simulink model "LTS_GGV"  (R2024b)
settings: Solver=ode4  StartTime=0.0  StopTime=5  FixedStep=0.001  RelTol=1e-3
values from neighbouring files (symbols this model uses):
  Accelcmd = 0    [generate_GGV_LTS_GGV.m]
  Decelcmd = Brk    [generate_GGV_LTS_GGV.m]
  Omega0 = V0/Rw    [generate_GGV_LTS_GGV.m]
  Steer_rad = deg2rad(SteerDeg)    [generate_GGV_LTS_GGV.m]
libraries: autolibsharedcoupling x1, vehdynlibsteering x1, autolibmappedmotor x1, autolibshared x1
(part 1 of 2)
settings Model: Creator=ASUS  LastModifiedBy=ASUS
settings DataIOCC: SaveState=on  InspectSignalLogs=on

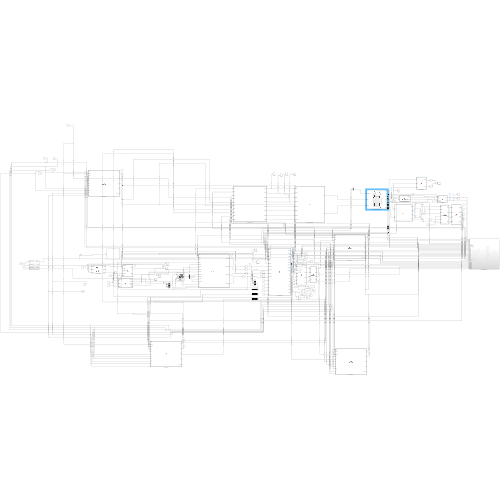
[thumbnail: Simulink's stored preview of the top-level diagram]
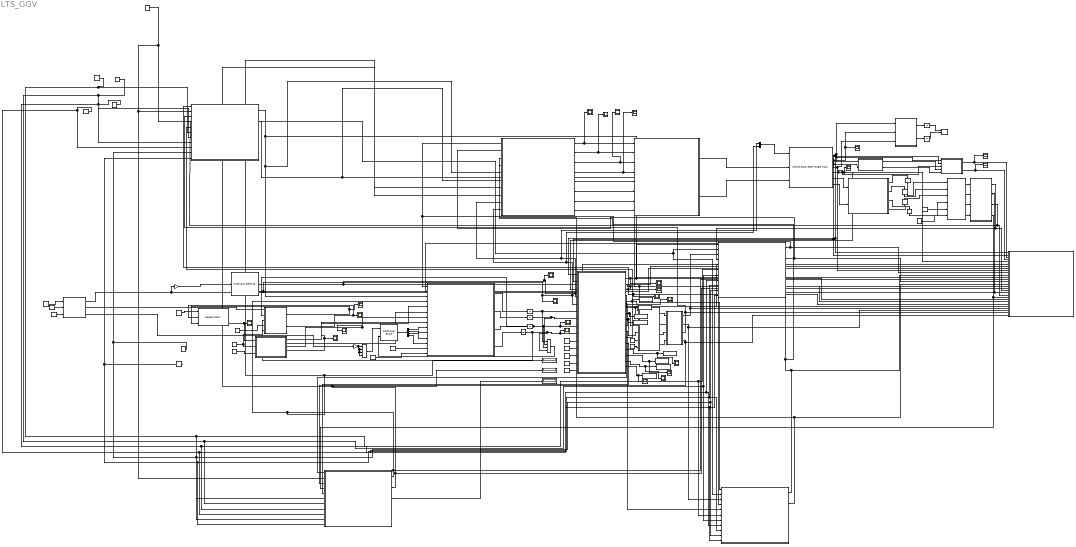
== system LTS_GGV ==
  "Accelaration " : MATLAB Function  TreatAsAtomicUnit=on
  Bodytoworld : MATLAB Function  TreatAsAtomicUnit=on
  Constant : Constant  Value=Steer_rad
  Constant1 : Constant  Value=0.10
  Constant10 : Constant  Value=0.001
  Constant11 : Constant  Value=0.08
  Constant12 : Constant  Value=0.03
  Constant13 : Constant  Value=0.001
  Constant14 : Constant  Value=Decelcmd
  Constant16 : Constant  Value=0.3
  Constant2 : Constant  Value=0.08
  Constant21 : Constant  Value=60
  Constant22 : Constant  Value=6
  Constant23 : Constant  Value=0.95
  Constant24 : Constant
  Constant3 : Constant  Value=0.30
  Constant31 : Constant  Value=0.8
  Constant32 : Constant  Value=0.8
  Constant33 : Constant  Value=1.2
  Constant34 : Constant  Value=1.2
  Constant35 : Constant  Value=0.3
  Constant4 : Constant
  Constant5 : Constant  Value=2.25e6
  Constant6 : Constant  Value=200
  Constant7 : Constant  Value=0
  Constant8 : Constant  Value=Accelcmd
  Constant9 : Constant
  Demux : Demux
  Disc Brake : autolibsharedcoupling/Rotational Brake  BrakeType=Disc  rotType=No inertia  extInfo=off  Iyy=1  br=1e-3  omegao=0  mu_static=0.4  mu_kinetic=0.35  disk_abore=0.02  Rm=0.08  num_pads=2  drum_abore=0.0508  drum_a=0.123  drum_c=0.212  drum_r=0.15  drum_theta1=0  drum_theta2=126  brake_p_bpt=[1 11.4736842105263 21.9473684210526 32.4210526315789 42.8947368421053 53.3684210526316 63.8421052631579 74.3157894736842 84.7894736842105 95.2631578947368 105.736842105263 116.210526315789 126.684210526316 137.157894736842 147.631578947368 158.105263157895 168.578947368421 179.052631578947 189.526315789474 200]  brake_n_bpt=[0 52.6315789473684 105.263157894737 157.894736842105 210.526315789474 263.157894736842 315.789473684211 368.421052631579 421.052631578947 473.684210526316 526.315789473684 578.947368421053 631.578947368421 684.210526315789 736.842105263158 789.473684210526 842.105263157895 894.736842105263 947.368421052632 1000]  f_brake_t=[43.4900602404453 42.5056030554862 41.5350898940194 40.5780454442085 39.6340111501808 38.7025443887544 37.7832176914519 36.8756180088306 35.9793460143796 35.0940154454303 34.2192524787115 33.3546951383474 32.4999927342521 31.6548053290159 30.8188032315107 29.991666515561 29.1730845621415 28.362755623661 27.5603864089927 26.765691687993;498.991217495636 487.695866636631 476.560505099801 465.579679307235 454.748127933653 444.060772460445 433.51270824929 423.099196101319 412.81565427025 402.657650900201 392.620896861006 382.701238955775 372.894653477208 363.197240090814 353.605216024701 344.114910546964 334.722759712992 325.425301366216 316.219170376863 307.10109410434;954.492374750826 932.886130217776 911.585920305583 890.581313170261 869.862244717126 849.419000532136 829.242198807128 809.322774193808 789.651962526121 770.221286354971 751.0225412433 732.047782773203 713.289314220164 694.739674852612 676.391628817892 658.238154578366 640.272434863842 622.48784710877 604.877954344734 587.436496520688;1409.99353200602 1378.07639379892 1346.61133551136 1315.58294703329 1284.9763615006 1254.77722860383 1224.97168936497 1195.5463522863 1166.48827078199 1137.78492180974 1109.42418562559 1081.39432659063 1053.68397496312 1026.28210961441 999.178041611083 972.361398609768 945.822110014692 919.550392851325 893.536738312604 867.771898937035;1865.49468926121 1823.26665738007 1781.63675071715 1740.58458089631 1700.09047828407 1660.13545667552 1620.7011799228 1581.76993037878 1543.32457903786 1505.34855726451 1467.82583000789 1430.74087040806 1394.07863570608 1357.82454437621 1321.96445440427 1286.48464264117 1251.37178516554 1216.61293859388 1182.19552228048 1148.10730135338;2320.9958465164 2268.45692096121 2216.66216592293 2165.58621475934 2115.20459506754 2065.49368474721 2016.43067048064 1967.99350847127 1920.16088729373 1872.91219271928 1826.22747439018 1780.08741422549 1734.47329644903 1689.36697913801 1644.75086719747 1600.60788667257 1556.92146031639 1513.67548433643 1470.85430624835 1428.44270376973;2776.49700377159 2713.64718454235 2651.68758112871 2590.58784862237 2530.31871185102 2470.8519128189 2412.16016103848 2354.21708656376 2296.9971955496 2240.47582817405 2184.62911877248 2129.43395804292 2074.86795719199 2020.9094138998 1967.53727999066 1914.73113070398 1862.47113546724 1810.73803007899 1759.51309021622 1708.77810618608;3231.99816102678 3158.8374481235 3086.71299633449 3015.58948248539 2945.43282863449 2876.21014089059 2807.88965159632 2740.44066465625 2673.83350380547 2608.03946362882 2543.03076315477 2478.78050186034 2415.26261793494 2352.4518486616 2290.32369278385 2228.85437473538 2168.02081061809 2107.80057582154 2048.17187418409 1989.11350860242;3687.49931828197 3604.02771170464 3521.73841154027 3440.59111634842 3360.54694541796 3281.56836896228 3203.61914215416 3126.66424274874 3050.66981206134 2975.60309908359 2901.43240753707 2828.12704567777 2755.6572786779 2683.9942834234 2613.11010557704 2542.97761876678 2473.57048576894 2404.8631215641 2336.83065815196 2269.44891101877;4143.00047553716 4049.21797528579 3956.76382674606 3865.59275021144 3775.66106220143 3686.92659703397 3599.34863271199 3512.88782084123 3427.50612031721 3343.16673453836 3259.83405191936 3177.4735894952 3096.05193942085 3015.5367181852 2935.89651837023 2857.10086279818 2779.12016091979 2701.92566730665 2625.48944211983 2549.78431343512;4598.50163279235 4494.40823886693 4391.78924195184 4290.59438407447 4190.77517898491 4092.28482510566 3995.07812326983 3899.11139893372 3804.34242857308 3710.73036999313 3618.23569630166 3526.82013331263 3436.44660016381 3347.079152947 3258.68293116342 3171.22410682959 3084.66983607064 2998.98821304921 2914.1482260877 2830.11971585147;5054.00279004754 4939.59850244808 4826.81465715762 4715.59601793749 4605.88929576838 4497.64305317735 4390.80761382767 4285.3349770262 4181.17873682896 4078.2940054479 3976.63734068395 3876.16667713006 3776.84126090677 3678.62158770879 3581.46934395661 3485.34735086099 ...(+2764 chars)]  aMode=2
      settings: LibrarySourceBlock=vehdynlibbrake/Disc Brake
  Display5 : Display
  Display6 : Display
  Display7 : Display
  "Force FWF and FWR " : MATLAB Function  TreatAsAtomicUnit=on
  Front_Left_tire : MATLAB Function  TreatAsAtomicUnit=on
  Front_Right_Tire : MATLAB Function  TreatAsAtomicUnit=on
  GGV Measurement : Subsystem
  Gain : Gain  Gain=8e+6
  Gain1 : Gain
  Integrator{,1..2,4} (4 alike) : Integrator  InitialCondition=Omega0
  Integrator3 : Integrator
  Integrator5 : Integrator
  Kinematic Steering : vehdynlibsteering/Kinematic Steering  StrgType=Ackerman  StrgRatioType=Constant  Loc=Front  NrmlFctr=0.01  TrckWdth=1.2  WhlBase=1.6  Db=0  StrgRng=deg2rad(25)  StrgAngBpts="[-6.2832   -5.0265   -3.7699   -2.5133   -1.2566         0    1.2566    2.5133    3.7699    5.0265    6.2832]"  StrgRatioTbl=|  StrgRatio=1  PctAckIn=off  PctAck=100  PctAckTbl=ones(1,11)*100  StrgArmLngth=0.1  RckCsLngth=0.5  TieRodLngth=0.248  D=0.2  PnnRadius=0.00085818  PnnRadiusTbl="[0.0055    0.0055    0.0056    0.0057    0.0058    0.0057    0.0057    0.0057    0.0056    0.0055    0.0055]"  RodLngth=0.1  ParaArmLngth=0.9  aMode=2
      | [13.5000   13.3750   13.2500   13.1250   13.0000   13.0000   13.0000   13.1250   13.2500   13.3750   13.5000
      | ]
  MATLAB Function : MATLAB Function  TreatAsAtomicUnit=on
  MATLAB Function1 : MATLAB Function  TreatAsAtomicUnit=on
  MATLAB Function2 : MATLAB Function  TreatAsAtomicUnit=on
  MATLAB Function3 : MATLAB Function  TreatAsAtomicUnit=on  SystemSampleTime=0.001
  MATLAB Function4 : MATLAB Function  TreatAsAtomicUnit=on
  MATLAB Function5 : MATLAB Function  TreatAsAtomicUnit=on  SystemSampleTime=0.001
  MATLAB Function6 : MATLAB Function  TreatAsAtomicUnit=on
  MATLAB Function7 : MATLAB Function  TreatAsAtomicUnit=on
  Mapped Motor : autolibmappedmotor/Mapped Motor  w_Tmax_bp_ext=w_Tmax_bp  Tmax_w_V_ext=Tmax_w_V  w_Tmin_bp_ext=w_Tmin_bp  Tmin_w_V_ext=Tmin_w_V  port_config=Speed  param_by=Maximum torque and power  w_t=[ 0 375 750 800 ]  T_t=[0.09 0.08 0.07 0]  torque_max=60  power_max=35000  SpreadsheetTqLimitsFileName=MotorCalibrationImportData.xlsx  Tmax_w_V=[0.09 0.09 0.09;0.08 0.08 0.08;0.07 0.07 0.07;0 0 0]  w_Tmax_bp=[ 0 375 750 800 ]  V_Tmax_bp=[500 750 900]  Tmin_w_V=[-0.09 -0.09 -0.09;-0.08 -0.08 -0.08;-0.07 -0.07 -0.07;0 0 0]  w_Tmin_bp=[ 0 375 750 800 ]  V_Tmin_bp=[500 750 900]  Tc=0.02  param_loss=Single efficiency measurement  SpreadsheetLossFileName=MotorCalibrationImportData.xlsx  SpreadsheetEffFileName=MotorCalibrationImportData.xlsx  eff=100  w_eff=375  T_eff=0.08  Piron=0  Pbase=0  w_eff_bp=[-8000 -4000 0 4000 8000]  T_eff_bp=[0 0.03 0.06 0.09]  Temp_eff_bp=[233.15 293.15 373.15]  V_eff_bp=[500 700 900]  losses_table=[1.49 1.67 2.21 3.10; 0.42 0.69 1.14 2.03; 0.06 0.24 0.78 1.68; 0.42 0.69 1.14 2.03; 1.49 1.67 2.21 3.10]  losses_table_3d=cat(3,1.05*[1.49 1.67 2.21 3.10; 0.42 0.69 1.14 2.03; 0.06 0.24 0.78 1.68; 0.42 0.69 1.14 2.03; 1.49 1.67 2.21 3.10],[1.49 1.67 2.21 3.10; 0.42 0.69 1.14 2.03; 0.06 0.24 0.78 1.68; 0.42 0.69 1.14 2.03; 1.49 1.67 2.21 3.10],1.03*[1.49 1.67 2.21 3.10; 0.42 0.69 1.14 2.03; 0.06 0.24 0.78 1.68; 0.42 0.69 1.14 2.03; 1.49 1.67 2.21 3.10])  losses_table_4d=cat(4,cat(3,[1.5645 0.441 0.063 0.441 1.5645;1.7535 0.7245 0.252 0.7245 1.7535;2.3205 1.197 0.819 1.197 2.3205;3.255 2.1315 1.764 2.1315 3.255],[1.5645 0.441 0.063 0.441 1.5645;1.7535 0.7245 0.252 0.7245 1.7535;2.3205 1.197 0.819 1.197 2.3205;3.255 2.1315 1.764 2.1315 3.255],[1.5645 0.441 0.063 0.441 1.5645;1.7535 0.7245 0.252 0.7245 1.7535;2.3205 1.197 0.819 1.197 2.3205;3.255 2.1315 1.764 2.1315 3.255]),cat(3,[1.49 0.42 0.06 0.42 1.49;1.67 0.69 0.24 0.69 1.67;2.21 1.14 0.78 1.14 2.21;3.1 2.03 1.68 2.03 3.1],[1.49 0.42 0.06 0.42 1.49;1.67 0.69 0.24 0.69 1.67;2.21 1.14 0.78 1.14 2.21;3.1 2.03 1.68 2.03 3.1],[1.49 0.42 0.06 0.42 1.49;1.67 0.69 0.24 0.69 1.67;2.21 1.14 0.78 1.14 2.21;3.1 2.03 1.68 2.03 3.1]),cat(3,[1.5347 0.4326 0.0618 0.4326 1.5347;1.7201 0.7107 0.2472 0.7107 1.7201;2.2763 1.1742 0.8034 1.1742 2.2763;3.193 2.0909 1.7304 2.0909 3.193],[1.5347 0.4326 0.0618 0.4326 1.5347;1.7201 0.7107 0.2472 0.7107 1.7201;2.2763 1.1742 0.8034 1.1742 2.2763;3.193 2.0909 1.7304 2.0909 3.193],[1.5347 0.4326 0.0618 0.4326 1.5347;1.7201 0.7107 0.2472 0.7107 1.7201;2.2763 1.1742 0.8034 1.1742 2.2763;3.193 2.0909 1.7304 2.0909 3.193]))  efficiency_table=[95 95 95 95; 95 95 95 95; 95 95 95 95; 95 95 95 95; 95 95 95 95]  efficiency_table_3d=cat(3,90*ones(5,4),95*ones(5,4),92*ones(5,4))  efficiency_table_4d=cat(4,cat(3,90*ones(5,4)',90*ones(5,4)',90*ones(5,4)'),cat(3,95*ones(5,4)',95*ones(5,4)',95*ones(5,4)'),cat(3,92*ones(5,4)',92*ones(5,4)',92*ones(5,4)'))  J=5e-6  b=1e-5  omega_o=0  T_t_extended=[0 0.07 0.08 0.09 0.08 0.07 0]  w_t_extended=[-800 -750 -375 0 375 750 800]  KLossIron=0  KLossCopper=0  x_w_eff_vec=[-8000 -4000 0 4000 8000]  x_T_eff_vec=[-0.09 -0.06 -0.03 0 0.03 0.06 0.09]  x_tmp_eff_vec=[233.15 293.15 373.15]  x_V_eff_vec=[500 700 900]  x_losses_mat=[3.1 2.21 1.67 1.49 1.67 2.21 3.1;2.03 1.14 0.69 0.42 0.69 1.14 2.03;1.68 0.78 0.24 0.06 0.24 0.78 1.68;2.03 1.14 0.69 0.42 0.69 1.14 2.03;3.1 2.21 1.67 1.49 1.67 2.21 3.1]  x_losses_mat_3d=cat(3,[3.255 2.3205 1.7535 1.5645 1.7535 2.3205 3.255;2.1315 1.197 0.7245 0.441 0.7245 1.197 2.1315;1.764 0.819 0.252 0.063 0.252 0.819 1.764;2.1315 1.197 0.7245 0.441 0.7245 1.197 2.1315;3.255 2.3205 1.7535 1.5645 1.7535 2.3205 3.255],[3.1 2.21 1.67 1.49 1.67 2.21 3.1;2.03 1.14 0.69 0.42 0.69 1.14 2.03;1.68 0.78 0.24 0.06 0.24 0.78 1.68;2.03 1.14 0.69 0.42 0.69 1.14 2.03;3.1 2.21 1.67 1.49 1.67 2.21 3.1],[3.193 2.2763 1.7201 1.5347 1.7201 2.2763 3.193;2.0909 1.1742 0.7107 0.4326 0.7107 1.1742 2.0909;1.7304 0.8034 0.2472 0.0618 0.2472 0.8034 1.7304;2.0909 1.1742 0.7107 0.4326 0.7107 1.1742 2.0909;3.193 2.2763 1.7201 1.5347 1.7201 2.2763 3.193])  x_losses_mat_4d=cat(4,cat(3,[1.5645 0.441 0.063 0.441 1.5645;1.7535 0.7245 0.252 0.7245 1.7535;2.3205 1.197 0.819 1.197 2.3205;3.255 2.1315 1.764 2.1315 3.255],[1.5645 0.441 0.063 0.441 1.5645;1.7535 0.7245 0.252 0.7245 1.7535;2.3205 1.197 0.819 1.197 2.3205;3.255 2.1315 1.764 2.1315 3.255],[1.5645 0.441 0.063 0.441 1.5645;1.7535 0.7245 0.252 0.7245 1.7535;2.3205 1.197 0.819 1.197 2.3205;3.255 2.1315 1.764 2.1315 3.255]),cat(3,[1.49 0.42 0.06 0.42 1.49;1.67 0.69 0.24 0.69 1.67;2.21 1.14 0.78 1.14 2.21;3.1 2.03 1.68 2.03 3.1],[1.49 0.42 0.06 0.42 1.49;1.67 0.69 0.24 0.69 1.67;2.21 1.14 0.78 1.14 2.21;3.1 2.03 1.68 2.03 3.1],[1.49 0.42 0.06 0.42 1.49;1.67 0.69 0.24 0.69 1.67;2.21 1.14 0.78 1.14 2.21;3.1 2.03 1.68 2.03 3.1]),cat(3,[1.5347 0.4326 0.0618 0.4326 1.5347;1.7201 0.7107 0.2472 0.7107 1.7201;2.2763 1.1742 0.8034 1.1742 2.2763;3.193 2.0909 1.7304 2.0909 3.193],[1.5347 0.4326 0.0618 0.4326 1.5347;1.7201 0.7107 0.2472 0.7107 1.7201;2.2763 1.1742 0.8034 1.1742 2.2763;3.193 2.0909 1.7304 2.0909 3.193],[1.5347 0.4326 0.0618 0.4326 1.5347;1.7201 0.7107 0.2472 0.7107 1.7201;2.2763 1.1742 0.8034 1.1742 2.2763;3.193 2.0909 1.7304 2.0909 3.193]))  CalLossMapData={}  CalLossWithTempMapData={}  aMode=2  RefBlkName='autolibmappedmotor/Mapped Motor'
      settings: LibrarySourceBlock=vdynlib/Powertrain/Propulsion/Mapped Motor
  Memory{,1..3} (4 alike) : Memory  InitialCondition=735.38
  Motor torque : Scope
  Mtr speed : Scope
  Mux : Mux  Inputs=2
  Omega RL : Scope
  Omega RR : Scope
  R : Scope
  "Rear_left tire " : MATLAB Function  TreatAsAtomicUnit=on
  Rear_right_tire : MATLAB Function  TreatAsAtomicUnit=on
  Scope{,1..9} (10 alike) : Scope
  Subsystem : Subsystem
  Tdrive RL : Scope
  Tdrive RR : Scope
  To Workspace1 : ToWorkspace  VariableName=VywFL  SampleTime=-1
      settings: Decimation=10
  To Workspace2 : ToWorkspace  VariableName=VxwFR  SampleTime=-1
      settings: Decimation=10
  To Workspace27 : ToWorkspace  VariableName=VxwFL  SampleTime=-1
      settings: Decimation=10
  To Workspace3 : ToWorkspace  VariableName=VywFR  SampleTime=-1
      settings: Decimation=10
  To Workspace4 : ToWorkspace  VariableName=kappaFL  SampleTime=-1
      settings: Decimation=10
  To Workspace5 : ToWorkspace  VariableName=kappaFR  SampleTime=-1
      settings: Decimation=10
  To Workspace6 : ToWorkspace  VariableName=kappaRL  SampleTime=-1
      settings: Decimation=10
  To Workspace7 : ToWorkspace  VariableName=kappaRR  SampleTime=-1
      settings: Decimation=10
  Trq commmand : Scope
  UY : Scope
  Vector Concatenate : Concatenate  NumInputs=4
  Vector Concatenate1 : Concatenate  NumInputs=4
  Vehicle Body 3DOF Dual Track : autolibshared/Vehicle Body 3DOF Single Track  trackMode=Dual  inputMode=External forces  frontSteerMode=on  rearSteerMode=off  windMode=off  muMode=off  extFMode=off  extMMode=off  htchFMode=off  htchMMode=off  extXo=off  extpsio=off  extxdoto=off  extro=off  extYo=off  extTamb=off  extydoto=off  aMode=2  NF=2  NR=2  m=300  a=0.8  b=0.8  h=0.3  dh=1  hh=0.2  X_o=0  xdot_o=V0  CalphaMode=off  sigmaMode=on  d=0  hl=0  w=[1.2,1.2]  Cy_f=12e3  Cy_r=11e3  sigma_f=.1  sigma_r=.1  alpha_f_brk=[-.1 .1]  Cy_f_data=[-9e3 9e3]  alpha_r_brk=[-.1 .1]  Cy_r_data=[-9e3 9e3]  Y_o=0  ydot_o=0  Izz=120  psi_o=0  r_o=0  Af=0  Cd=0  Cl=0  Cpm=0  beta_w=[0 0.01:0.01:0.3]  Cs=[0:0.03:0.9]  Cym=[0 1e-6:0.01:0.3]  Pabs=101325  Tair=273  g=9.81  mu=1  xdot_tol=.01  Fznom=5000  Fxtire_sat=7e4  Fytire_sat=7e4  longOff=0  latOff=0  vertOff=0  wrapAng=off
      settings: LibrarySourceBlock=vehdynlibeom/Vehicle Body 3DOF Dual Track
  VehicleVelocityDerivative : MATLAB Function  TreatAsAtomicUnit=on
  Wheel kinematics : MATLAB Function  TreatAsAtomicUnit=on
  XY Graph : Record  FileSettingsInternal="{\"entries\":[{\"content\":{\"excelSettings\":{\"content\":{},\"type\":\"Streamout.ExcelSettings\"}},\"type\":\"Streamout.FileSettingStorage\",\"uuid\":\"\"}],\"packageUris\":[\"http:\\/\\/schema.mathworks.com\\/mf0\\/streamout_blocks\\/R2020a\"],\"version\":\"1.0\"}"  Layout=[1 1]  SignalsInternal="{\"entries\":[{\"content\":{\"signals\":[{\"content\":{\"blockPath\":[],\"dimensions\":[1],\"domain\":\"\",\"lineColor\":\"#edb120\",\"lineWidth\":2,\"port\":1,\"sid\":[\"\"],\"signalID\":1,\"signalName\":\"X_sim\"},\"type\":\"RecordBlkView.Signal\",\"uuid\":\"\"},{\"content\":{\"blockPath\":[],\"dimensions\":[1],\"domain\":\"\",\"lineColor\":\"#7e2f8e\",\"lineWidth\":2,\"port\":2,\"sid\":[\"\"],\"signalID\":2,\"signalName\":\"Y_sim\"},\"type\":\"RecordBlkView.Signal\",\"uuid\":\"\"}]},\"type\":\"RecordBlkView.InputSignals\",\"uuid\":\"\"}],\"packageUris\":[\"http:\\/\\/schema.mathworks.com\\/mf0\\/streamout_blocks\\/R2020a\"],\"version\":\"1.0\"}"  VisualizationBindings="{\"xyplotplugin\":{\"info\":[{\"series\":[],\"subplotID\":1}]}}"  CompatibilityTag=XY
  fx fl : Scope
  fxfr : Scope
  fyfl : Scope
  fyfr : Scope
  "left angle " : Scope
  "right angle " : Scope
  "wheel to vehicle " : MATLAB Function  TreatAsAtomicUnit=on
  wires:
  Mux/1 -> Vehicle Body 3DOF Dual Track/1
  Integrator4/1 -> Vector Concatenate/4, Omega RR/1, Wheel kinematics/9(omegaRR), MATLAB Function6/3(omegaRR)
  MATLAB Function4/1(kFLs) -> GGV Measurement/26(KappaFL), Front_Left_tire/3(kappa)
  "Force FWF and FWR "/2(FwR) -> Vehicle Body 3DOF Dual Track/3
  Vehicle Body 3DOF Dual Track/7 -> MATLAB Function/2(FzR)
  Integrator2/1 -> Omega RL/1, Wheel kinematics/8(omegaRL), Vector Concatenate/3, MATLAB Function6/2(omegaRL)
  MATLAB Function4/2(kFRs) -> GGV Measurement/27(KappaFR), Front_Right_Tire/3(kappa)
  MATLAB Function4/3(kRLs) -> GGV Measurement/28(KappaRL), "Rear_left tire "/3(kappa)
  MATLAB Function4/4(kRRs) -> GGV Measurement/29(KappaRR), Rear_right_tire/3(kappa)
  Integrator/1 -> Vector Concatenate/1, Wheel kinematics/6(omegaFL)
  Vehicle Body 3DOF Dual Track/4 -> Bodytoworld/3(psi), GGV Measurement/9(PSI)
  Vehicle Body 3DOF Dual Track/3 -> "Accelaration "/2(ydot), Bodytoworld/2(ydot), UY/1, Wheel kinematics/2(Uy), GGV Measurement/2(Vy), VehicleVelocityDerivative/2(Uy)
  Vehicle Body 3DOF Dual Track/2 -> VehicleVelocityDerivative/1(Ux), "Accelaration "/1(xdot), Bodytoworld/1(xdot), GGV Measurement/1(Vx), Wheel kinematics/1(Ux)
  Vehicle Body 3DOF Dual Track/5 -> "Accelaration "/3(r), Wheel kinematics/3(r), R/1, GGV Measurement/5(r)
  Vehicle Body 3DOF Dual Track/6 -> MATLAB Function/1(FzF)
  Kinematic Steering/3 -> GGV Measurement/8(front-right steer), "right angle "/1, Wheel kinematics/5(deltaFR), Mux/2, "wheel to vehicle "/10(deltaFR)
  Front_Left_tire/2(Fy) -> "wheel to vehicle "/2(FyFL), GGV Measurement/14(FyFL)
  "wheel to vehicle "/4(FyVehFR) -> fyfr/1, "Force FWF and FWR "/4(FyVehFR)
  Constant6/1 -> "Rear_left tire "/11(n), Front_Right_Tire/11(n), Front_Left_tire/11(n), Rear_right_tire/11(n)
  Rear_right_tire/2(Fy) -> GGV Measurement/17(FyRR), Display6/1, "wheel to vehicle "/8(FyRR)
  Constant16/1 -> MATLAB Function1/13(Rw)
  Wheel kinematics/12(VcRR) -> Rear_right_tire/5(Vc)
  Constant34/1 -> Wheel kinematics/13(tr)
  Integrator1/1 -> Vector Concatenate/2, Wheel kinematics/7(omegaFR)
  Constant5/1 -> Front_Left_tire/10(cp), Front_Right_Tire/10(cp), Rear_right_tire/10(cp), "Rear_left tire "/10(cp)
  MATLAB Function1/2(omegaDotFR) -> Integrator1/1
  Front_Right_Tire/2(Fy) -> GGV Measurement/15(FyFR), "wheel to vehicle "/4(FyFR)
  "Rear_left tire "/1(Fx) -> GGV Measurement/12(FxRL), MATLAB Function1/3(FxRL), "wheel to vehicle "/5(FxRL)
  Constant35/1 -> Wheel kinematics/14(Rw)
  Constant32/1 -> Wheel kinematics/11(lr)
  MATLAB Function1/4(omegaDotRR) -> Integrator4/1
  Front_Right_Tire/1(Fx) -> GGV Measurement/11(FxFR), MATLAB Function1/2(FxFR), "wheel to vehicle "/3(FxFR)
  Constant3/1 -> "Rear_left tire "/8(re), Front_Left_tire/8(re), Front_Right_Tire/8(re), Rear_right_tire/8(re)
  "wheel to vehicle "/6(FyVehRL) -> "Force FWF and FWR "/6(FyVehRL)
  Wheel kinematics/9(VcFL) -> Front_Left_tire/5(Vc)
  Constant4/1 -> "Rear_left tire "/9(mu0), Front_Left_tire/9(mu0), Front_Right_Tire/9(mu0), Rear_right_tire/9(mu0)
  Constant7/1 -> Front_Right_Tire/2(gamma), Front_Left_tire/2(gamma), Rear_right_tire/2(gamma), "Rear_left tire "/2(gamma)
  "wheel to vehicle "/1(FxVehFL) -> fx fl/1, "Force FWF and FWR "/1(FxVehFL)
  "wheel to vehicle "/3(FxVehFR) -> fxfr/1, "Force FWF and FWR "/3(FxVehFR)
  Rear_right_tire/3(Mz) -> Display7/1
  Front_Left_tire/1(Fx) -> GGV Measurement/10(FxFL), MATLAB Function1/1(FxFL), "wheel to vehicle "/1(FxFL)
  MATLAB Function1/1(omegaDotFL) -> Integrator/1
  Wheel kinematics/3(alphaRL) -> Scope2/1, GGV Measurement/24(AlphaRL), "Rear_left tire "/1(alpha)
  Rear_right_tire/1(Fx) -> GGV Measurement/13(FxRR), MATLAB Function1/4(FxRR), Display5/1, "wheel to vehicle "/7(FxRR)
  Constant1/1 -> "Rear_left tire "/6(a), Front_Left_tire/6(a), Front_Right_Tire/6(a), Rear_right_tire/6(a)
  Wheel kinematics/11(VcRL) -> "Rear_left tire "/5(Vc)
  Kinematic Steering/2 -> GGV Measurement/7(front-left steer), Wheel kinematics/4(deltaFL), Mux/1, "wheel to vehicle "/9(deltaFL), "left angle "/1
  Constant31/1 -> Wheel kinematics/10(lf)
  MATLAB Function1/3(omegaDotRL) -> Integrator2/1
  Wheel kinematics/4(alphaRR) -> Scope3/1, GGV Measurement/25(AlphaRR), Rear_right_tire/1(alpha)
  "wheel to vehicle "/5(FxVehRL) -> "Force FWF and FWR "/5(FxVehRL)
  Wheel kinematics/1(alphaFL) -> Scope/1, GGV Measurement/22(AlphaFL), Front_Left_tire/1(alpha)
  Constant2/1 -> "Rear_left tire "/7(b), Front_Left_tire/7(b), Front_Right_Tire/7(b), Rear_right_tire/7(b)
  Wheel kinematics/10(VcFR) -> Front_Right_Tire/5(Vc)
  "wheel to vehicle "/8(FyVehRR) -> "Force FWF and FWR "/8(FyVehRR)
  Constant33/1 -> Wheel kinematics/12(tf)
  Constant9/1 -> MATLAB Function1/14(Iw)
  "wheel to vehicle "/7(FxVehRR) -> "Force FWF and FWR "/7(FxVehRR)
  "wheel to vehicle "/2(FyVehFL) -> fyfl/1, "Force FWF and FWR "/2(FyVehFL)
  Wheel kinematics/2(alphaFR) -> Scope1/1, GGV Measurement/23(AlphaFR), Front_Right_Tire/1(alpha)
  "Rear_left tire "/2(Fy) -> GGV Measurement/16(FyRL), "wheel to vehicle "/6(FyRL)
  "Force FWF and FWR "/1(FwF) -> Vehicle Body 3DOF Dual Track/2
  MATLAB Function/4(FzRR) -> Memory3/1
  MATLAB Function/1(FzFL) -> Memory/1
  MATLAB Function/2(FzFR) -> Memory2/1
  MATLAB Function/3(FzRL) -> Memory1/1
  Memory/1 -> MATLAB Function2/1(FzFL)
  Memory1/1 -> MATLAB Function2/3(FzRL)
  Memory2/1 -> MATLAB Function2/2(FzFR)
  Memory3/1 -> MATLAB Function2/4(FzRR)
  MATLAB Function3/3(FzRLs) -> "Rear_left tire "/4(Fz), GGV Measurement/20(FzRL)
  MATLAB Function3/1(FzFLs) -> GGV Measurement/18(FzFL), Front_Left_tire/4(Fz)
  MATLAB Function3/2(FzFRs) -> GGV Measurement/19(FzFR), Front_Right_Tire/4(Fz)
  MATLAB Function3/4(FzRRs) -> Rear_right_tire/4(Fz), GGV Measurement/21(FzRR)
  Constant10/1 -> MATLAB Function2/5(dt)
  Constant11/1 -> MATLAB Function2/6(tau)
  MATLAB Function2/1(FzFLf) -> MATLAB Function3/1(FzFL)
  MATLAB Function2/2(FzFRf) -> MATLAB Function3/2(FzFR)
  MATLAB Function2/3(FzRLf) -> MATLAB Function3/3(FzRL)
  MATLAB Function2/4(FzRRf) -> MATLAB Function3/4(FzRR)
  Wheel kinematics/8(kappaRR) -> To Workspace7/1, MATLAB Function5/4(kRR)
  Wheel kinematics/6(kappaFR) -> To Workspace5/1, MATLAB Function5/2(kFR)
  Wheel kinematics/5(kappaFL) -> To Workspace4/1, MATLAB Function5/1(kFL)
  Disc Brake/1 -> Demux/1
  MATLAB Function5/1(kFLf) -> MATLAB Function4/1(kFL)
  MATLAB Function5/2(kFRf) -> MATLAB Function4/2(kFR)
  MATLAB Function5/3(kRLf) -> MATLAB Function4/3(kRL)
  MATLAB Function5/4(kRRf) -> MATLAB Function4/4(kRR)
  Constant12/1 -> MATLAB Function5/6(tau)
  Constant13/1 -> MATLAB Function5/5(dt)
  Mapped Motor/3 -> MATLAB Function7/1(MtrTrq), Motor torque/1
  Constant21/1 -> MATLAB Function6/4(TmotorMax)
  Constant22/1 -> MATLAB Function7/2(Ndiff), MATLAB Function6/5(Ndiff)
  Constant23/1 -> MATLAB Function7/3(etaDiff)
  MATLAB Function6/1(TrqCmd) -> Mapped Motor/3, Trq commmand/1
  MATLAB Function6/2(MtrSpd) -> Mtr speed/1, Mapped Motor/2
  Constant24/1 -> Mapped Motor/1
  MATLAB Function7/1(TdriveFL) -> MATLAB Function1/5(TdriveFL)
  MATLAB Function7/2(TdriveFR) -> MATLAB Function1/6(TdriveFR)
  MATLAB Function7/3(TdriveRL) -> MATLAB Function1/7(TdriveRL), Tdrive RL/1
  MATLAB Function7/4(TdriveRR) -> MATLAB Function1/8(TdriveRR), Tdrive RR/1
  Vector Concatenate/1 -> Disc Brake/2
  Gain/1 -> Vector Concatenate1/4, Vector Concatenate1/3, Vector Concatenate1/2, Vector Concatenate1/1
  Vector Concatenate1/1 -> Disc Brake/1
  Demux/1 -> MATLAB Function1/9(TbrakeFL)
  Demux/2 -> MATLAB Function1/10(TbrakeFR)
  Demux/3 -> MATLAB Function1/11(TbrakeRL)
  Demux/4 -> MATLAB Function1/12(TbrakeRR)
  Bodytoworld/1(Xdot_w) -> Integrator3/1
  Bodytoworld/2(Ydot_w) -> Integrator5/1
  Integrator3/1 -> XY Graph/1  "X_sim"
  Integrator5/1 -> XY Graph/2  "Y_sim"
  Gain1/1 -> Kinematic Steering/1
  VehicleVelocityDerivative/1(Ux_dot) -> "Accelaration "/4(xdot_deriv)
  VehicleVelocityDerivative/2(Uy_dot) -> "Accelaration "/5(ydot_deriv)
  "Accelaration "/2(ay_G) -> Scope9/1, GGV Measurement/4(Ay)
  "Accelaration "/1(ax_G) -> Scope8/1, GGV Measurement/3(Ax)
  Subsystem/1(SteerCmd) -> GGV Measurement/6(steer_cmd), Gain1/1
  Subsystem/2(Accel) -> MATLAB Function6/1(throttleCmd)
  Subsystem/3(Decel) -> Gain/1
  Wheel kinematics/13(VxwFL) -> Scope4/1, To Workspace27/1
  Wheel kinematics/14(VywFL) -> Scope5/1, To Workspace1/1
  Wheel kinematics/15(VxwFR) -> Scope6/1, To Workspace2/1
  Wheel kinematics/16(VywFR) -> Scope7/1, To Workspace3/1
  Constant/1 -> Subsystem/1(" SteerCmd_GGV")
  Constant8/1 -> Subsystem/2(AccelCmd_GGV)
  Constant14/1 -> Subsystem/3(DecelCmd_GGV)
  Wheel kinematics/7(kappaRL) -> To Workspace6/1, MATLAB Function5/3(kRL)

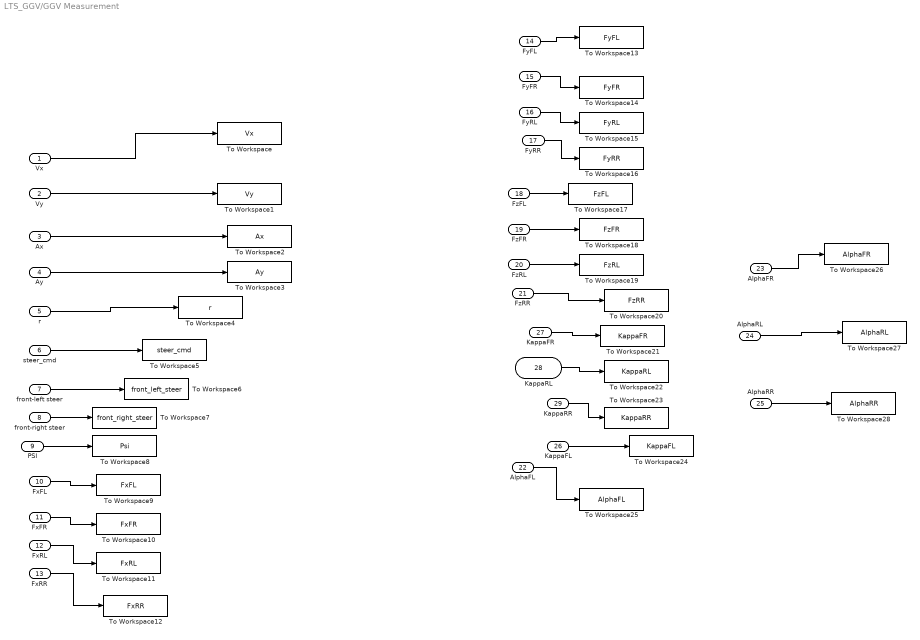
== system LTS_GGV/GGV Measurement ==
  Vx : Inport
  Vy : Inport  Port=2
  Ax : Inport  Port=3
  Ay : Inport  Port=4
  r : Inport  Port=5
  steer_cmd : Inport  Port=6
  front-left steer : Inport  Port=7
  front-right steer : Inport  Port=8
  PSI : Inport  Port=9
  FxFL : Inport  Port=10
  FxFR : Inport  Port=11
  FxRL : Inport  Port=12
  FxRR : Inport  Port=13
  FyFL : Inport  Port=14
  FyFR : Inport  Port=15
  FyRL : Inport  Port=16
  FyRR : Inport  Port=17
  FzFL : Inport  Port=18
  FzFR : Inport  Port=19
  FzRL : Inport  Port=20
  FzRR : Inport  Port=21
  AlphaFL : Inport  Port=22
  AlphaFR : Inport  Port=23
  AlphaRL : Inport  Port=24
  AlphaRR : Inport  Port=25
  KappaFL : Inport  Port=26
  KappaFR : Inport  Port=27
  KappaRL : Inport  Port=28
  KappaRR : Inport  Port=29
  To Workspace : ToWorkspace  VariableName=Vx  SampleTime=-1
      settings: Decimation=10
  To Workspace1 : ToWorkspace  VariableName=Vy  SampleTime=-1
      settings: Decimation=10
  To Workspace10 : ToWorkspace  VariableName=FxFR  SampleTime=-1
      settings: Decimation=10
  To Workspace11 : ToWorkspace  VariableName=FxRL  SampleTime=-1
      settings: Decimation=10
  To Workspace12 : ToWorkspace  VariableName=FxRR  SampleTime=-1
      settings: Decimation=10
  To Workspace13 : ToWorkspace  VariableName=FyFL  SampleTime=-1
      settings: Decimation=10
  To Workspace14 : ToWorkspace  VariableName=FyFR  SampleTime=-1
      settings: Decimation=10
  To Workspace15 : ToWorkspace  VariableName=FyRL  SampleTime=-1
      settings: Decimation=10
  To Workspace16 : ToWorkspace  VariableName=FyRR  SampleTime=-1
      settings: Decimation=10
  To Workspace17 : ToWorkspace  VariableName=FzFL  SampleTime=-1
      settings: Decimation=10
  To Workspace18 : ToWorkspace  VariableName=FzFR  SampleTime=-1
      settings: Decimation=10
  To Workspace19 : ToWorkspace  VariableName=FzRL  SampleTime=-1
      settings: Decimation=10
  To Workspace2 : ToWorkspace  VariableName=Ax  SampleTime=-1
      settings: Decimation=10
  To Workspace20 : ToWorkspace  VariableName=FzRR  SampleTime=-1
      settings: Decimation=10
  To Workspace21 : ToWorkspace  VariableName=KappaFR  SampleTime=-1
      settings: Decimation=10
  To Workspace22 : ToWorkspace  VariableName=KappaRL  SampleTime=-1
      settings: Decimation=10
  To Workspace23 : ToWorkspace  VariableName=KappaRR  SampleTime=-1
      settings: Decimation=10
  To Workspace24 : ToWorkspace  VariableName=KappaFL  SampleTime=-1
      settings: Decimation=10
  To Workspace25 : ToWorkspace  VariableName=AlphaFL  SampleTime=-1
      settings: Decimation=10
  To Workspace26 : ToWorkspace  VariableName=AlphaFR  SampleTime=-1
      settings: Decimation=10
  To Workspace27 : ToWorkspace  VariableName=AlphaRL  SampleTime=-1
      settings: Decimation=10
  To Workspace28 : ToWorkspace  VariableName=AlphaRR  SampleTime=-1
      settings: Decimation=10
  To Workspace3 : ToWorkspace  VariableName=Ay  SampleTime=-1
      settings: Decimation=10
  To Workspace4 : ToWorkspace  VariableName=r  SampleTime=-1
      settings: Decimation=10
  To Workspace5 : ToWorkspace  VariableName=steer_cmd  SampleTime=-1
      settings: Decimation=10
  To Workspace6 : ToWorkspace  VariableName=front_left_steer  SampleTime=-1
      settings: Decimation=10
  To Workspace7 : ToWorkspace  VariableName=front_right_steer  SampleTime=-1
      settings: Decimation=10
  To Workspace8 : ToWorkspace  VariableName=Psi  SampleTime=-1
      settings: Decimation=10
  To Workspace9 : ToWorkspace  VariableName=FxFL  SampleTime=-1
      settings: Decimation=10
  wires:
  Vx/1 -> To Workspace/1
  Vy/1 -> To Workspace1/1
  Ax/1 -> To Workspace2/1
  Ay/1 -> To Workspace3/1
  r/1 -> To Workspace4/1
  steer_cmd/1 -> To Workspace5/1
  front-left steer/1 -> To Workspace6/1
  front-right steer/1 -> To Workspace7/1
  PSI/1 -> To Workspace8/1
  FxFL/1 -> To Workspace9/1
  FxFR/1 -> To Workspace10/1
  FxRL/1 -> To Workspace11/1
  FxRR/1 -> To Workspace12/1
  FyFL/1 -> To Workspace13/1
  FyFR/1 -> To Workspace14/1
  FyRL/1 -> To Workspace15/1
  FyRR/1 -> To Workspace16/1
  FzFL/1 -> To Workspace17/1
  FzFR/1 -> To Workspace18/1
  FzRL/1 -> To Workspace19/1
  FzRR/1 -> To Workspace20/1
  KappaFR/1 -> To Workspace21/1
  KappaRL/1 -> To Workspace22/1
  KappaRR/1 -> To Workspace23/1
  KappaFL/1 -> To Workspace24/1
  AlphaFL/1 -> To Workspace25/1
  AlphaFR/1 -> To Workspace26/1
  AlphaRL/1 -> To Workspace27/1
  AlphaRR/1 -> To Workspace28/1

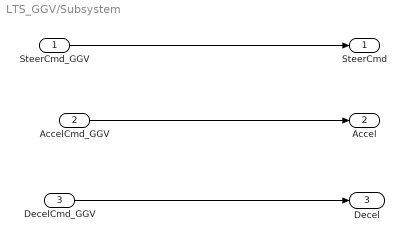
== system LTS_GGV/Subsystem ==
  " SteerCmd_GGV" : Inport
  AccelCmd_GGV : Inport  Port=2
  DecelCmd_GGV : Inport  Port=3
  SteerCmd : Outport
  Accel : Outport  Port=2
  Decel : Outport  Port=3
  wires:
  DecelCmd_GGV/1 -> Decel/1
  AccelCmd_GGV/1 -> Accel/1
  " SteerCmd_GGV"/1 -> SteerCmd/1

== matlab function LTS_GGV/Rear_right_tire ==
  data: alpha input; Fx output; gamma input; kappa input; Fz input; Vc input; a input; b input; re input; mu0 input; cp input; n input; Fy output; Mz output; Mx output; slide_count output
function [Fx,Fy,Mz,Mx,slide_count] = tread_model( ...
                alpha,...
                gamma,...
                kappa,...
                Fz,...
                Vc,...
                a,b,re,...
                mu0,...
                cp,...
                n)

%%%%%%%%%%%%%%%%%%%%%%%%%%%%%%%%%%%%%%%%%%%%%%%%%%%%%%%%%%%%
% CONTACT PATCH
%%%%%%%%%%%%%%%%%%%%%%%%%%%%%%%%%%%%%%%%%%%%%%%%%%%%%%%%%%%%

xb = linspace(a,-a,n);

dx = abs(xb(2)-xb(1));

%%%%%%%%%%%%%%%%%%%%%%%%%%%%%%%%%%%%%%%%%%%%%%%%%%%%%%%%%%%%
% ROLLING KINEMATICS
%%%%%%%%%%%%%%%%%%%%%%%%%%%%%%%%%%%%%%%%%%%%%%%%%%%%%%%%%%%%

Vr = Vc/(1-kappa);

Omega = Vr/re;

dt = dx/Vr;

%%%%%%%%%%%%%%%%%%%%%%%%%%%%%%%%%%%%%%%%%%%%%%%%%%%%%%%%%%%%
% SLIP VELOCITIES
%%%%%%%%%%%%%%%%%%%%%%%%%%%%%%%%%%%%%%%%%%%%%%%%%%%%%%%%%%%%

Vsx = -Vc*kappa;

Vsy = -Vc*tan(alpha);

%%%%%%%%%%%%%%%%%%%%%%%%%%%%%%%%%%%%%%%%%%%%%%%%%%%%%%%%%%%%
% MULTI ROW TREAD
%%%%%%%%%%%%%%%%%%%%%%%%%%%%%%%%%%%%%%%%%%%%%%%%%%%%%%%%%%%%

nRows = 11;

yrow = linspace(-b,b,nRows);

dyrow = (2*b)/(nRows-1);

%%%%%%%%%%%%%%%%%%%%%%%%%%%%%%%%%%%%%%%%%%%%%%%%%%%%%%%%%%%%
% OUTPUT INITIALIZATION
%%%%%%%%%%%%%%%%%%%%%%%%%%%%%%%%%%%%%%%%%%%%%%%%%%%%%%%%%%%%

Fx = 0;
Fy = 0;
Mz = 0;
Mx = 0;

slide_count = 0;

%%%%%%%%%%%%%%%%%%%%%%%%%%%%%%%%%%%%%%%%%%%%%%%%%%%%%%%%%%%%
% PRESSURE NORMALIZATION
%%%%%%%%%%%%%%%%%%%%%%%%%%%%%%%%%%%%%%%%%%%%%%%%%%%%%%%%%%%%

ShapeSum = 0;

for r = 1:nRows

    yb0 = yrow(r);

    for i = 1:n

        px = max(0,1-(xb(i)/a)^2);

        py = sqrt(max(0,1-(yb0/b)^2));

        ShapeSum = ShapeSum + px*py*dx*dyrow;

    end
end

qz0 = Fz/ShapeSum;

%%%%%%%%%%%%%%%%%%%%%%%%%%%%%%%%%%%%%%%%%%%%%%%%%%%%%%%%%%%%
% MAIN LOOP
%%%%%%%%%%%%%%%%%%%%%%%%%%%%%%%%%%%%%%%%%%%%%%%%%%%%%%%%%%%%

for r = 1:nRows

    yb0 = yrow(r);

    ex = 0;
    ey = 0;

    for i = 1:n

        px = max(0,1-(xb(i)/a)^2);

        py = sqrt(max(0,1-(yb0/b)^2));

        qz = qz0*px*py;

        if qz <= 0
            continue
        end

        dybdx = (xb(i)/re)*sin(gamma);

        Vbx = Vsx + yb0*Omega*sin(gamma);

        Vby = Vsy - Vr*dybdx;

        %%%%%%%%%%%%%%%%%%%%%%%%%%%%%%%%%%%%%%%%%%%%%%%%%%%%
        % CONSTANT FRICTION
        %%%%%%%%%%%%%%%%%%%%%%%%%%%%%%%%%%%%%%%%%%%%%%%%%%%%

        qlimit = mu0*qz;

        Dsx = Vbx*dt;

        Dsy = Vby*dt;

        ex_trial = ex - Dsx;

        ey_trial = ey - Dsy;

        qx_trial = cp*ex_trial;

        qy_trial = cp*ey_trial;

        qtrial = hypot(qx_trial,qy_trial);

        %%%%%%%%%%%%%%%%%%%%%%%%%%%%%%%%%%%%%%%%%%%%%%%%%%%%
        % ADHESION
        %%%%%%%%%%%%%%%%%%%%%%%%%%%%%%%%%%%%%%%%%%%%%%%%%%%%

        if qtrial <= qlimit

            ex = ex_trial;
            ey = ey_trial;

            qx = cp*ex;
            qy = cp*ey;

        %%%%%%%%%%%%%%%%%%%%%%%%%%%%%%%%%%%%%%%%%%%%%%%%%%%%
        % SLIDING
        %%%%%%%%%%%%%%%%%%%%%%%%%%%%%%%%%%%%%%%%%%%%%%%%%%%%

        else

            slide_count = slide_count + 1;

            e_i = qlimit/cp;

            norm_trial = hypot(ex_trial,ey_trial);

            if norm_trial > 1e-12

                ex = e_i*ex_trial/norm_trial;

                ey = e_i*ey_trial/norm_trial;

            else

                ex = 0;
                ey = 0;

            end

            qx = cp*ex;
            qy = cp*ey;

        end

        dA = dx*dyrow;

        dFx = qx*dA;
        dFy = qy*dA;

        Fx = Fx + dFx;
        Fy = Fy + dFy;

        Mz = Mz + xb(i)*dFy - yb0*dFx;

        Mx = Mx + yb0*dFy;

    end
end

end

== matlab function LTS_GGV/Front_Right_Tire ==
  data: alpha input; Fx output; gamma input; kappa input; Fz input; Vc input; a input; b input; re input; mu0 input; cp input; n input; Fy output; Mz output; Mx output; slide_count output
function [Fx,Fy,Mz,Mx,slide_count] = tread_model( ...
                alpha,...
                gamma,...
                kappa,...
                Fz,...
                Vc,...
                a,b,re,...
                mu0,...
                cp,...
                n)

%%%%%%%%%%%%%%%%%%%%%%%%%%%%%%%%%%%%%%%%%%%%%%%%%%%%%%%%%%%%
% CONTACT PATCH
%%%%%%%%%%%%%%%%%%%%%%%%%%%%%%%%%%%%%%%%%%%%%%%%%%%%%%%%%%%%

xb = linspace(a,-a,n);

dx = abs(xb(2)-xb(1));

%%%%%%%%%%%%%%%%%%%%%%%%%%%%%%%%%%%%%%%%%%%%%%%%%%%%%%%%%%%%
% ROLLING KINEMATICS
%%%%%%%%%%%%%%%%%%%%%%%%%%%%%%%%%%%%%%%%%%%%%%%%%%%%%%%%%%%%

Vr = Vc/(1-kappa);

Omega = Vr/re;

dt = dx/Vr;

%%%%%%%%%%%%%%%%%%%%%%%%%%%%%%%%%%%%%%%%%%%%%%%%%%%%%%%%%%%%
% SLIP VELOCITIES
%%%%%%%%%%%%%%%%%%%%%%%%%%%%%%%%%%%%%%%%%%%%%%%%%%%%%%%%%%%%

Vsx = -Vc*kappa;

Vsy = -Vc*tan(alpha);

%%%%%%%%%%%%%%%%%%%%%%%%%%%%%%%%%%%%%%%%%%%%%%%%%%%%%%%%%%%%
% MULTI ROW TREAD
%%%%%%%%%%%%%%%%%%%%%%%%%%%%%%%%%%%%%%%%%%%%%%%%%%%%%%%%%%%%

nRows = 11;

yrow = linspace(-b,b,nRows);

dyrow = (2*b)/(nRows-1);

%%%%%%%%%%%%%%%%%%%%%%%%%%%%%%%%%%%%%%%%%%%%%%%%%%%%%%%%%%%%
% OUTPUT INITIALIZATION
%%%%%%%%%%%%%%%%%%%%%%%%%%%%%%%%%%%%%%%%%%%%%%%%%%%%%%%%%%%%

Fx = 0;
Fy = 0;
Mz = 0;
Mx = 0;

slide_count = 0;

%%%%%%%%%%%%%%%%%%%%%%%%%%%%%%%%%%%%%%%%%%%%%%%%%%%%%%%%%%%%
% PRESSURE NORMALIZATION
%%%%%%%%%%%%%%%%%%%%%%%%%%%%%%%%%%%%%%%%%%%%%%%%%%%%%%%%%%%%

ShapeSum = 0;

for r = 1:nRows

    yb0 = yrow(r);

    for i = 1:n

        px = max(0,1-(xb(i)/a)^2);

        py = sqrt(max(0,1-(yb0/b)^2));

        ShapeSum = ShapeSum + px*py*dx*dyrow;

    end
end

qz0 = Fz/ShapeSum;

%%%%%%%%%%%%%%%%%%%%%%%%%%%%%%%%%%%%%%%%%%%%%%%%%%%%%%%%%%%%
% MAIN LOOP
%%%%%%%%%%%%%%%%%%%%%%%%%%%%%%%%%%%%%%%%%%%%%%%%%%%%%%%%%%%%

for r = 1:nRows

    yb0 = yrow(r);

    ex = 0;
    ey = 0;

    for i = 1:n

        px = max(0,1-(xb(i)/a)^2);

        py = sqrt(max(0,1-(yb0/b)^2));

        qz = qz0*px*py;

        if qz <= 0
            continue
        end

        dybdx = (xb(i)/re)*sin(gamma);

        Vbx = Vsx + yb0*Omega*sin(gamma);

        Vby = Vsy - Vr*dybdx;

        %%%%%%%%%%%%%%%%%%%%%%%%%%%%%%%%%%%%%%%%%%%%%%%%%%%%
        % CONSTANT FRICTION
        %%%%%%%%%%%%%%%%%%%%%%%%%%%%%%%%%%%%%%%%%%%%%%%%%%%%

        qlimit = mu0*qz;

        Dsx = Vbx*dt;

        Dsy = Vby*dt;

        ex_trial = ex - Dsx;

        ey_trial = ey - Dsy;

        qx_trial = cp*ex_trial;

        qy_trial = cp*ey_trial;

        qtrial = hypot(qx_trial,qy_trial);

        %%%%%%%%%%%%%%%%%%%%%%%%%%%%%%%%%%%%%%%%%%%%%%%%%%%%
        % ADHESION
        %%%%%%%%%%%%%%%%%%%%%%%%%%%%%%%%%%%%%%%%%%%%%%%%%%%%

        if qtrial <= qlimit

            ex = ex_trial;
            ey = ey_trial;

            qx = cp*ex;
            qy = cp*ey;

        %%%%%%%%%%%%%%%%%%%%%%%%%%%%%%%%%%%%%%%%%%%%%%%%%%%%
        % SLIDING
        %%%%%%%%%%%%%%%%%%%%%%%%%%%%%%%%%%%%%%%%%%%%%%%%%%%%

        else

            slide_count = slide_count + 1;

            e_i = qlimit/cp;

            norm_trial = hypot(ex_trial,ey_trial);

            if norm_trial > 1e-12

                ex = e_i*ex_trial/norm_trial;

                ey = e_i*ey_trial/norm_trial;

            else

                ex = 0;
                ey = 0;

            end

            qx = cp*ex;
            qy = cp*ey;

        end

        dA = dx*dyrow;

        dFx = qx*dA;
        dFy = qy*dA;

        Fx = Fx + dFx;
        Fy = Fy + dFy;

        Mz = Mz + xb(i)*dFy - yb0*dFx;

        Mx = Mx + yb0*dFy;

    end
end

end

== matlab function LTS_GGV/wheel to vehicle  ==
  data: FxFL input; FxVehFL output; FyFL input; FxFR input; FyFR input; FxRL input; FyRL input; FxRR input; FyRR input; deltaFL input; deltaFR input; FyVehFL output; FxVehFR output; FyVehFR output; FxVehRL output; FyVehRL output; FxVehRR output; FyVehRR output
function [FxVehFL,FyVehFL,FxVehFR,FyVehFR, ...
          FxVehRL,FyVehRL,FxVehRR,FyVehRR] = TransformForces( ...
          FxFL,FyFL,FxFR,FyFR, ...
          FxRL,FyRL,FxRR,FyRR, ...
          deltaFL,deltaFR)
%#codegen

% Front-left wheel frame to vehicle frame
FxVehFL = FxFL*cos(deltaFL) - FyFL*sin(deltaFL);
FyVehFL = -FxFL*sin(deltaFL) + FyFL*cos(deltaFL);

% Front-right wheel frame to vehicle frame
FxVehFR = FxFR*cos(deltaFR) - FyFR*sin(deltaFR);
FyVehFR = -FxFR*sin(deltaFR) + FyFR*cos(deltaFR);

% Rear wheels are not steered
FxVehRL = FxRL;
FyVehRL = FyRL;

FxVehRR = FxRR;
FyVehRR = FyRR;

end

== matlab function LTS_GGV/Force FWF and FWR  ==
  data: FxVehFL input; FwF output; FyVehFL input; FxVehFR input; FyVehFR input; FxVehRL input; FyVehRL input; FxVehRR input; FyVehRR input; FwR output
function [FwF,FwR] = BuildForceInputs( ...
    FxVehFL,FyVehFL,FxVehFR,FyVehFR, ...
    FxVehRL,FyVehRL,FxVehRR,FyVehRR)
%#codegen

% Correct Vehicle Body 3DOF format:
% Row 1 = left wheel
% Row 2 = right wheel
% Column 1 = Fx
% Column 2 = Fy

FwF = [FxVehFL  FyVehFL;
       FxVehFR  FyVehFR];

FwR = [FxVehRL  FyVehRL;
       FxVehRR  FyVehRR];

end

== matlab function LTS_GGV/MATLAB Function ==
  data: FzF input; FzFL output; FzR input; FzFR output; FzRL output; FzRR output
function [FzFL,FzFR,FzRL,FzRR] = SplitFz(FzF,FzR)
%#codegen

FzFL = 0.0;
FzFR = 0.0;
FzRL = 0.0;
FzRR = 0.0;

% Linear indexing works for both row and column vectors
FzFL = FzF(1);
FzFR = FzF(2);

FzRL = FzR(1);
FzRR = FzR(2);

end

== matlab function LTS_GGV/MATLAB Function1 ==
  data: FxFL input; omegaDotFL output; FxFR input; FxRL input; FxRR input; TdriveFL input; TdriveFR input; TdriveRL input; TdriveRR input; TbrakeFL input; TbrakeFR input; TbrakeRL input; TbrakeRR input; Rw input; Iw input; omegaDotFR output; omegaDotRL output; omegaDotRR output
function [omegaDotFL,omegaDotFR,omegaDotRL,omegaDotRR] = WheelDynamics( ...
    FxFL,FxFR,FxRL,FxRR, ...
    TdriveFL,TdriveFR,TdriveRL,TdriveRR, ...
    TbrakeFL,TbrakeFR,TbrakeRL,TbrakeRR, ...
    Rw,Iw)

omegaDotFL = 0.0;
omegaDotFR = 0.0;
omegaDotRL = 0.0;
omegaDotRR = 0.0;

omegaDotFL = (TdriveFL - TbrakeFL - FxFL*Rw)/Iw;
omegaDotFR = (TdriveFR - TbrakeFR - FxFR*Rw)/Iw;
omegaDotRL = (TdriveRL - TbrakeRL - FxRL*Rw)/Iw;
omegaDotRR = (TdriveRR - TbrakeRR - FxRR*Rw)/Iw;

end

== matlab function LTS_GGV/MATLAB Function2 ==
  data: FzFL input; FzFLf output; FzFR input; FzRL input; FzRR input; dt input; tau input; FzFRf output; FzRLf output; FzRRf output
function [FzFLf,FzFRf,FzRLf,FzRRf] = FzLowPass( ...
    FzFL,FzFR,FzRL,FzRR,dt,tau)
%#codegen

persistent zFL zFR zRL zRR initialized

if isempty(initialized)
    zFL = FzFL;
    zFR = FzFR;
    zRL = FzRL;
    zRR = FzRR;
    initialized = true;
end

alpha = dt/(tau + dt);

zFL = zFL + alpha*(FzFL - zFL);
zFR = zFR + alpha*(FzFR - zFR);
zRL = zRL + alpha*(FzRL - zRL);
zRR = zRR + alpha*(FzRR - zRR);

FzFLf = zFL;
FzFRf = zFR;
FzRLf = zRL;
FzRRf = zRR;

end

== matlab function LTS_GGV/MATLAB Function3 ==
  data: FzFL input; FzFLs output; FzFR input; FzRL input; FzRR input; FzFRs output; FzRLs output; FzRRs output
function [FzFLs,FzFRs,FzRLs,FzRRs] = FzSafety(FzFL,FzFR,FzRL,FzRR)
%#codegen

FzMin = 50.0;

FzFLs = max(FzFL,FzMin);
FzFRs = max(FzFR,FzMin);
FzRLs = max(FzRL,FzMin);
FzRRs = max(FzRR,FzMin);

end

== matlab function LTS_GGV/MATLAB Function4 ==
  data: kFL input; kFLs output; kFR input; kRL input; kRR input; kFRs output; kRLs output; kRRs output
function [kFLs,kFRs,kRLs,kRRs] = KappaSafety(kFL,kFR,kRL,kRR)


kMin = -0.30;
kMax =  0.30;

kFLs = min(max(kFL,kMin),kMax);
kFRs = min(max(kFR,kMin),kMax);
kRLs = min(max(kRL,kMin),kMax);
kRRs = min(max(kRR,kMin),kMax);

end

== matlab function LTS_GGV/MATLAB Function5 ==
  data: kFL input; kFLf output; kFR input; kRL input; kRR input; dt input; tau input; kFRf output; kRLf output; kRRf output
function [kFLf,kFRf,kRLf,kRRf] = KappaLowPass(kFL,kFR,kRL,kRR,dt,tau)
%#codegen

persistent zFL zFR zRL zRR initialized

if isempty(initialized)
    zFL = kFL;
    zFR = kFR;
    zRL = kRL;
    zRR = kRR;
    initialized = true;
end

alpha = dt/(tau + dt);

zFL = zFL + alpha*(kFL - zFL);
zFR = zFR + alpha*(kFR - zFR);
zRL = zRL + alpha*(kRL - zRL);
zRR = zRR + alpha*(kRR - zRR);

kFLf = zFL;
kFRf = zFR;
kRLf = zRL;
kRRf = zRR;

end

== matlab function LTS_GGV/MATLAB Function6 ==
  data: throttleCmd input; TrqCmd output; omegaRL input; omegaRR input; TmotorMax input; Ndiff input; MtrSpd output
function [TrqCmd, MtrSpd] = EV_Command_And_Speed( ...
    throttleCmd, omegaRL, omegaRR, TmotorMax, Ndiff)


%% Safe inputs
throttle = min(max(throttleCmd, 0.0), 1.0);
Tmax     = max(TmotorMax, 0.0);
N        = max(Ndiff, 0.01);

%% Throttle to motor torque request
TrqCmd = throttle*Tmax;

%% Open-differential speed relationship
omegaCarrier = 0.5*(omegaRL + omegaRR);
MtrSpd       = N*omegaCarrier;

end

== matlab function LTS_GGV/MATLAB Function7 ==
  data: MtrTrq input; TdriveFL output; Ndiff input; etaDiff input; TdriveFR output; TdriveRL output; TdriveRR output; Taxle output
function [TdriveFL, TdriveFR, TdriveRL, TdriveRR, Taxle] = ...
    Open_Differential_Torque(MtrTrq, Ndiff, etaDiff)


%% Safe parameters
N   = max(Ndiff, 0.01);
eta = min(max(etaDiff, 0.0), 1.0);

%% Total torque after reduction
Taxle = MtrTrq*N*eta;

%% Rear-wheel-drive configuration
TdriveFL = 0.0;
TdriveFR = 0.0;

%% Ideal open differential: equal wheel torque
TdriveRL = 0.5*Taxle;
TdriveRR = 0.5*Taxle;

end

== matlab function LTS_GGV/Bodytoworld ==
  data: xdot input; Xdot_w output; ydot input; psi input; Ydot_w output
function [Xdot_w, Ydot_w] = BodyToWorld(xdot, ydot, psi)

Xdot_w = xdot*cos(psi) - ydot*sin(psi);
Ydot_w = xdot*sin(psi) + ydot*cos(psi);

== matlab function LTS_GGV/VehicleVelocityDerivative ==
  settings: updateMethod=DISCRETE
  data: Ux input; Ux_dot output; Uy input; Uy_dot output
function [Ux_dot, Uy_dot] = VehicleVelocityDerivative(Ux, Uy)
%#codegen
%
% Discrete second-order backward derivative.
%
% Block sample time must be fixed at Ts = 0.01 s.
%
% Ux     : longitudinal body velocity [m/s]
% Uy     : lateral body velocity [m/s]
%
% Ux_dot : dUx/dt [m/s^2]
% Uy_dot : dUy/dt [m/s^2]

persistent Ux_1 Ux_2
persistent Uy_1 Uy_2
persistent initialized

Ts = 0.001;

if isempty(initialized)

    % Initialize history with the actual initial velocities.
    Ux_1 = Ux;
    Ux_2 = Ux;

    Uy_1 = Uy;
    Uy_2 = Uy;

    initialized = true;

    Ux_dot = 0;
    Uy_dot = 0;

    return;
end

% Second-order backward difference
Ux_dot = ...
    (3*Ux - 4*Ux_1 + Ux_2)/(2*Ts);

Uy_dot = ...
    (3*Uy - 4*Uy_1 + Uy_2)/(2*Ts);

% Update history
Ux_2 = Ux_1;
Ux_1 = Ux;

Uy_2 = Uy_1;
Uy_1 = Uy;

end

== matlab function LTS_GGV/Accelaration  ==
  data: xdot input; ax_G output; ydot input; r input; xdot_deriv input; ydot_deriv input; ay_G output
function [ax_G, ay_G] = calculate_GG(xdot, ydot, r, xdot_deriv, ydot_deriv)
    % Define gravity
    g = 9.80665; % m/s^2
    
    % Calculate true body-frame accelerations (m/s^2)
    % Accounting for centripetal acceleration (v * r)
    ax_mps2 = xdot_deriv - (ydot * r);
    ay_mps2 = ydot_deriv + (xdot * r);
    
    % Convert to G-Forces
    ax_G = ax_mps2 / g;
    ay_G = ay_mps2 / g;
end
